simulink library "INT_HLSDem_SetPoint"  (R2016b)
settings: Solver=VariableStepAuto  StartTime=0.0  StopTime=10.0  RelTol=1e-3
settings Model: Creator=xuxingpei  LastModifiedBy=xuxingpei

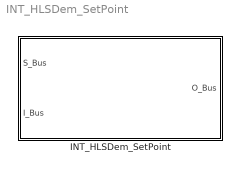
== system INT_HLSDem_SetPoint ==
  INT_HLSDem_SetPoint : Subsystem

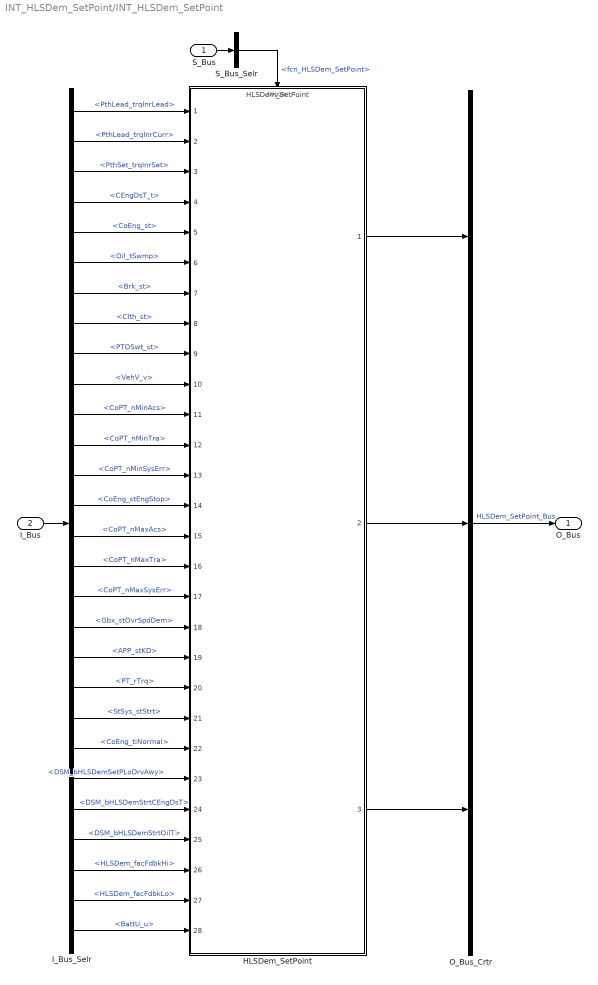
== system INT_HLSDem_SetPoint/INT_HLSDem_SetPoint ==
  S_Bus : Inport
  I_Bus : Inport  Port=2
  HLSDem_SetPoint : ModelReference  ModelNameDialog=HLSDem_SetPoint  SimulationMode=Normal  ModelReferenceVersion=1.119  TriggerPortName=function  TriggerPortTriggerType=function-call  TriggerPortStatesWhenEnabling=held
  I_Bus_Selr : BusSelector  OutputSignals=PthLead_trqInrLead,PthLead_trqInrCurr,PthSet_trqInrSet,CEngDsT_t,CoEng_st,Oil_tSwmp,Brk_st,Clth_st,PTOSwt_st,VehV_v,CoPT_nMinAcs,CoPT_nMinTra,CoPT_nMinSysErr,CoEng_stEngStop,CoPT_nMaxAcs,CoPT_nMaxTra,CoPT_nMaxSysErr,Gbx_stOvrSpdDem,APP_stKD,PT_rTrq,StSys_stStrt,CoEng_tiNormal,DSM_bHLSDemSetPLoDrvAwy,DSM_bHLSDemStrtCEngDsT,DSM_bHLSDemStrtOilT,HLSDem_facFdbkHi,HLSDem_facFdbkLo,BattU_u
  O_Bus_Crtr : BusCreator  Inputs=3
  S_Bus_Selr : BusSelector  OutputSignals=fcn_HLSDem_SetPoint
  O_Bus : Outport
  wires:
  S_Bus_Selr/1 -> HLSDem_SetPoint/Trigger  "<fcn_HLSDem_SetPoint>"
  S_Bus/1 -> S_Bus_Selr/1
  I_Bus/1 -> I_Bus_Selr/1
  I_Bus_Selr/1 -> HLSDem_SetPoint/1  "<PthLead_trqInrLead>"
  I_Bus_Selr/2 -> HLSDem_SetPoint/2  "<PthLead_trqInrCurr>"
  I_Bus_Selr/3 -> HLSDem_SetPoint/3  "<PthSet_trqInrSet>"
  I_Bus_Selr/4 -> HLSDem_SetPoint/4  "<CEngDsT_t>"
  I_Bus_Selr/5 -> HLSDem_SetPoint/5  "<CoEng_st>"
  I_Bus_Selr/6 -> HLSDem_SetPoint/6  "<Oil_tSwmp>"
  I_Bus_Selr/7 -> HLSDem_SetPoint/7  "<Brk_st>"
  I_Bus_Selr/8 -> HLSDem_SetPoint/8  "<Clth_st>"
  I_Bus_Selr/9 -> HLSDem_SetPoint/9  "<PTOSwt_st>"
  I_Bus_Selr/10 -> HLSDem_SetPoint/10  "<VehV_v>"
  I_Bus_Selr/11 -> HLSDem_SetPoint/11  "<CoPT_nMinAcs>"
  I_Bus_Selr/12 -> HLSDem_SetPoint/12  "<CoPT_nMinTra>"
  I_Bus_Selr/13 -> HLSDem_SetPoint/13  "<CoPT_nMinSysErr>"
  I_Bus_Selr/14 -> HLSDem_SetPoint/14  "<CoEng_stEngStop>"
  I_Bus_Selr/15 -> HLSDem_SetPoint/15  "<CoPT_nMaxAcs>"
  I_Bus_Selr/16 -> HLSDem_SetPoint/16  "<CoPT_nMaxTra>"
  I_Bus_Selr/17 -> HLSDem_SetPoint/17  "<CoPT_nMaxSysErr>"
  I_Bus_Selr/18 -> HLSDem_SetPoint/18  "<Gbx_stOvrSpdDem>"
  I_Bus_Selr/19 -> HLSDem_SetPoint/19  "<APP_stKD>"
  I_Bus_Selr/20 -> HLSDem_SetPoint/20  "<PT_rTrq>"
  I_Bus_Selr/21 -> HLSDem_SetPoint/21  "<StSys_stStrt>"
  I_Bus_Selr/22 -> HLSDem_SetPoint/22  "<CoEng_tiNormal>"
  I_Bus_Selr/23 -> HLSDem_SetPoint/23  "<DSM_bHLSDemSetPLoDrvAwy>"
  I_Bus_Selr/24 -> HLSDem_SetPoint/24  "<DSM_bHLSDemStrtCEngDsT>"
  I_Bus_Selr/25 -> HLSDem_SetPoint/25  "<DSM_bHLSDemStrtOilT>"
  I_Bus_Selr/26 -> HLSDem_SetPoint/26  "<HLSDem_facFdbkHi>"
  I_Bus_Selr/27 -> HLSDem_SetPoint/27  "<HLSDem_facFdbkLo>"
  I_Bus_Selr/28 -> HLSDem_SetPoint/28  "<BattU_u>"
  O_Bus_Crtr/1 -> O_Bus/1  "HLSDem_SetPoint_Bus"
  HLSDem_SetPoint/1 -> O_Bus_Crtr/1
  HLSDem_SetPoint/2 -> O_Bus_Crtr/2
  HLSDem_SetPoint/3 -> O_Bus_Crtr/3
